simulink model "rl_top_5_bus"  (Simulink 10.3)
settings: Solver=VariableStepAuto  StartTime=0.0  StopTime=1  RelTol=1e-3  EnableMultiTasking=on
model workspace (MAT data in the model file):
  agent5bus1 : rl.agent.rlDDPGAgent (value not decoded)
  linsys1 = ss
  linsys1.InputName_ = ["M1 200 MVA/1"; "M1 200 MVA/2"]
  linsys1.OutputName_ = ["M1 200 MVA/1(1)"; "M1 200 MVA/1(2)"; "M1 200 MVA/1(3)"; "M1 200 MVA/1(4)"; "M1 200 MVA/1(5)"; "M1 200 MVA/1(6)"; "M1 200 MVA/1(7)"; "M1 200 MVA/1(8)"; "M1 200 MVA/1(9)"; "M1 200 MVA/1(10)"; "M1 200 MVA/1(11)"; "M1 200 MVA/1(12)"; "M1 200 MVA/1(13)"; "M1 200 MVA/1(14)"; "M1 200 MVA/1(15)"; "M1 200 MVA/1(16)"; "M1 200 MVA/1(17)"; "M1 200 MVA/1(18)"; "M1 200 MVA/1(19)"; "M1 200 MVA/1(20)"; "M1 200 MVA/1(21)"; "M1 200 MVA/1(22)"; "M1 200 MVA/1(23)"; "M1 200 MVA/1(24)"]
  linsys1.Name_ = 'Linearization at model initial condition'
  linsys1.IOSize_ = [24 2]
  linsys1.Data_ = ltipack.ssdata
  linsys1.Data_.StateName = ["dw_delay"; "dw_predict"; "Rotor angle dthetae"; "Rotor speed deviation (dw)"; "theta"; "State-Space(1)"; "State-Space(2)"; "State-Space(3)"; "State-Space(4)"; "State-Space(5)"; "State-Space(6)"]
  linsys1.Data_.StatePath = ["untitled/M1 200 MVA/Mechanical model/Delay Prediction/dw_delay"; "untitled/M1 200 MVA/Mechanical model/Delay Prediction/dw_predict"; "untitled/M1 200 MVA/Mechanical model/Rotor angle dthetae"; "untitled/M1 200 MVA/Mechanical model/Rotor speed deviation (dw)"; "untitled/M1 200 MVA/Mechanical model/theta"; "untitled/powergui/EquivalentModel1/State-Space"; "untitled/powergui/EquivalentModel1/State-Space"; "untitled/powergui/EquivalentModel1/State-Space"; "untitled/powergui/EquivalentModel1/State-Space"; "untitled/powergui/EquivalentModel1/State-Space"; "untitled/powergui/EquivalentModel1/State-Space"]
  linsys1.Data_.a = [-5.58783784007e-05  2.79391892004e-05  0  1  0  0  0  0  0  0  0; 1  0  0  0  0  0  0  0  0  0  0; 0.376991118431  -0.188495559215  1  0  0  0  0  0  0  0  0; -0.000111756756801  5.58783784007e-05  0  1  0  0  0  0  0  0  0; 0.011780972451  -0.00589048622548  0  0  1  0  0  0  0  0  0; 0  0  26991.0065171  0  0  0.998213204856  2.92569216118e-09  0  0  0  0; 0  0  463941227454  0  0  -30712.746053  0.0502889439339  0  0  0  0; 0  0  -15831.6103638  0  0  0  0  0.998213204856  2.92569216479e-09  0  0; 0  0  -272125337019  0  0  0  0  -30712.7460413  0.0502889439331  0  0; 0  0  -11159.3961502  0  0  0  0  0  0  0.998213204873  2.92569216375e-09; 0  0  -191815890454  0  0  0  0  0  0  -30712.7459983  0.0502889439397]
  linsys1.Data_.b = [3.37837837838e-05  0; 0  0; 0  0; 6.75675675675e-05  0; 0  0; 0  0; 0  0; 0  0; 0  0; 0  0; 0  0]
  linsys1.Data_.c = [0  0  0.832534925644  0  0  0  0  0  0  0  0; 0  0  -0.488324455382  0  0  0  0  0  0  0  0; 0  0  -0.344210470262  0  0  0  0  0  0  0  0; 0  0  0  0  0  0  0  0  0  0  0; 0  0  0  0  0  0  0  0  0  0  0; 0  0  0  0  0  0  0  0  0  0  0; 0  0  0  0  0  0  0  0  0  0  0; 0  0  0  0  0  0  0  0  0  0  0; 0  0  0  0  0  0  0  0  0  0  0; 0  0  0  0  0  0  0  0  0  0  0; 0  0  0  0  0  0  0  0  0  0  0; 0  0  -431.358163988  0  0  -0.000282911073761  4.63237611855e-10  0.000692715872014  -1.1342505678e-09  -0.000409804798927  6.71012956118e-10; 0  0  757.168110723  0  0  0.000636540605551  -1.04226938184e-09  -7.32621253784e-05  1.1995915085e-10  -0.000563278480852  9.22310230491e-10; 0  0  0  0  0  0  0  0  0  0  0; 0  0  0  0  0  0  0  0  0  0  0; 0  0  1  0  0  0  0  0  0  0  0; 2  -1  0  0  0  0  0  0  0  0  0; 1.65399613714  -0.826998068568  0  0  0  0  0  0  0  0  0; 2  -1  0  0  0  0  0  0  0  0  0; 0  0  0  0  57.2957795131  0  0  0  0  0  0; 0  0  0  0  0  0  0  0  0  0  0; 0  0  2.98373081066  0  0  2.37325451245e-06  -3.88595871507e-12  -1.39203573926e-06  2.27931449655e-12  -9.81218774074e-07  1.60664421675e-12; 0  0  -0.0012497256202  0  0  5.79583507644e-05  -9.4900802709e-11  0.000473251935921  -7.74901079242e-10  -0.000531210287457  8.69801881873e-10; 0  0  -729.102017304  0  0  -0.000579926534214  9.49569697606e-10  0.000340156670938  -5.56971354471e-10  0.000239769863491  -3.925983427e-10]
  linsys1.Data_.d = [0  0; 0  0; 0  0; 0  0; 0  0; 0  0; 0  0; 0  0; 0  0; 0  0; 0  0; 0  0; 0  0; 0  0; 0  0; 0  0; 0  0; 0  0; 0  0; 0  0; 0  0; 0  0; 0  0; 0  0]
  linsys1.Data_.Delay.Input = [0; 0]
  linsys1.Data_.Delay.Output = [0; 0; 0; 0; 0; 0; 0; 0; 0; 0; 0; 0; 0; 0; 0; 0; 0; 0; 0; 0; 0; 0; 0; 0]
  linsys1.Data_.Delay.Internal = []
  linsys1.Data_.Ts = 0.0005
libraries: simulink x6, rllib x1
settings Model: Creator=Rodney Tan  LastModifiedBy=User
settings DataIOCC: SignalLoggingSaveFormat=Dataset  SignalLogging=off  DSMLogging=off
settings OptimizationCC: ExpressionDepthLimit=128
settings DebuggingCC: UnderspecifiedInitializationDetection=Simplified  MergeDetectMultiDrivingBlocksExec=error  FcnCallInpInsideContextMsg=error  UnconnectedInputMsg=none  UnconnectedOutputMsg=none  UnconnectedLineMsg=none  StateNameClashWarn=none  SFExecutionAtInitializationDiag=warning
settings HardwareCC: ProdBitPerPointer=64  ProdBitPerSizeT=64  ProdBitPerPtrDiffT=64  ProdLargestAtomicFloat=Float  ProdIntDivRoundTo=Zero  ProdEndianess=LittleEndian  ProdWordSize=64  ProdHWDeviceType=Intel->x86-64 (Windows64)
settings ModelReferenceCC: PropagateSignalLabelsOutOfModel=on
settings GRTTargetCC: CombineOutputUpdateFcns=on  GRTInterface=off
settings SimscapeCC: SimscapeNormalizeSystem=off

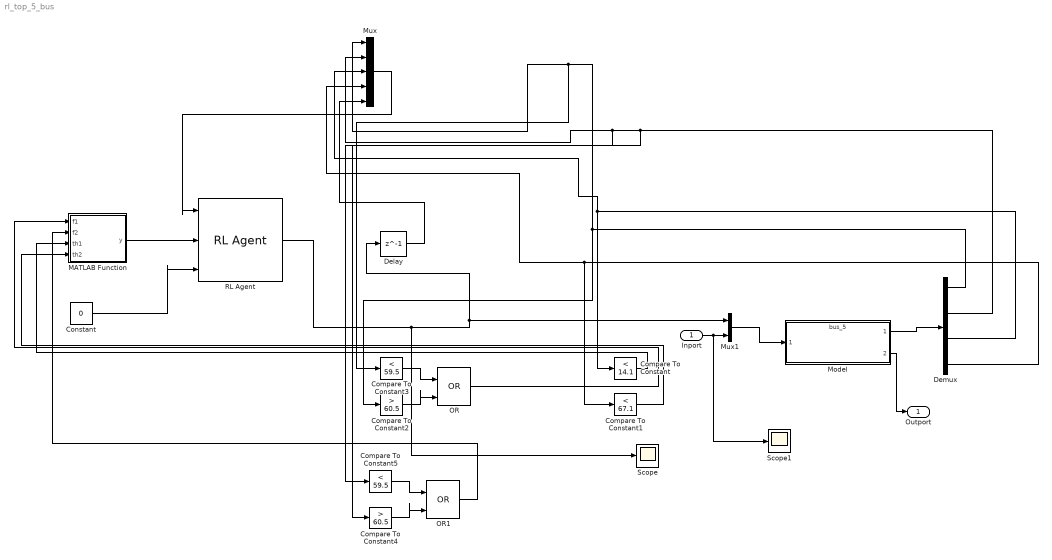
== system rl_top_5_bus ==
  Inport : Inport
  Compare To Constant : simulink/Logic and Bit Operations/Compare To Constant  relop=<  const=14.1  OutDataTypeStr=boolean
  Compare To Constant1 : simulink/Logic and Bit Operations/Compare To Constant  relop=<  const=67.1  OutDataTypeStr=boolean
  Compare To Constant2 : simulink/Logic and Bit Operations/Compare To Constant  relop=>  const=60.5  OutDataTypeStr=boolean
  Compare To Constant3 : simulink/Logic and Bit Operations/Compare To Constant  relop=<  const=59.5  OutDataTypeStr=boolean
  Compare To Constant4 : simulink/Logic and Bit Operations/Compare To Constant  relop=>  const=60.5  OutDataTypeStr=boolean
  Compare To Constant5 : simulink/Logic and Bit Operations/Compare To Constant  relop=<  const=59.5  OutDataTypeStr=boolean
  Constant : Constant  Value=0
  Delay : Delay  DelayLength=1
  Demux : Demux
  MATLAB Function : MATLAB Function  TreatAsAtomicUnit=on
  Model : ModelReference  ModelNameDialog=bus_5.mdl  SimulationMode=Normal  ModelReferenceVersion=1.20
  Mux : Mux  Inputs=5
  Mux1 : Mux  Inputs=2
  OR : Logic  Operator=OR  IconShape=distinctive  AllPortsSameDT=off  OutDataTypeStr=boolean
  OR1 : Logic  Operator=OR  IconShape=distinctive  AllPortsSameDT=off  OutDataTypeStr=boolean
  RL Agent : rllib/RL Agent  Agent=agent5bus1  ExternalActionAsInput=off  ProvideCumRwd=off  TreatAsDirectFeedthrough=on
  Scope : Scope
  Scope1 : Scope
  Outport : Outport
  wires:
  RL Agent/1 -> Scope/1, Mux1/1, Delay/1
  Demux/1 -> Compare To Constant3/1, Mux/1, Compare To Constant2/1
  Demux/3 -> Mux/3, Compare To Constant/1
  Demux/4 -> Compare To Constant1/1, Mux/4
  Mux/1 -> RL Agent/1
  Delay/1 -> Mux/5
  MATLAB Function/1(y) -> RL Agent/2
  Constant/1 -> RL Agent/3
  Compare To Constant3/1 -> OR/1
  Compare To Constant2/1 -> OR/2
  Demux/2 -> Compare To Constant4/1, Compare To Constant5/1, Mux/2
  Compare To Constant5/1 -> OR1/1
  Compare To Constant4/1 -> OR1/2
  OR/1 -> MATLAB Function/1(f1)
  OR1/1 -> MATLAB Function/2(f2)
  Compare To Constant/1 -> MATLAB Function/3(th1)
  Compare To Constant1/1 -> MATLAB Function/4(th2)
  Inport/1 -> Scope1/1, Mux1/2
  Mux1/1 -> Model/1
  Model/1 -> Demux/1
  Model/2 -> Outport/1

== matlab function MATLAB Function ==
  data: f1 input double; y output double; f2 input double; th1 input double; th2 input double
function y = fcn(f1, f2, th1, th2)
w1=7;
w2=5;
rwd= (w1*(f1*th1)+w2*(f2*th2));
y = rwd;
